simulink model "Example_7"  (R2020b)
settings: Solver=VariableStepAuto  StartTime=0.0  StopTime=0.1  RelTol=1e-3
libraries: fl_lib x10, nesl_utility x4, dspsigops x3, ee_lib x3
settings Model: Creator=zaliyazici  LastModifiedBy=zaliyazici

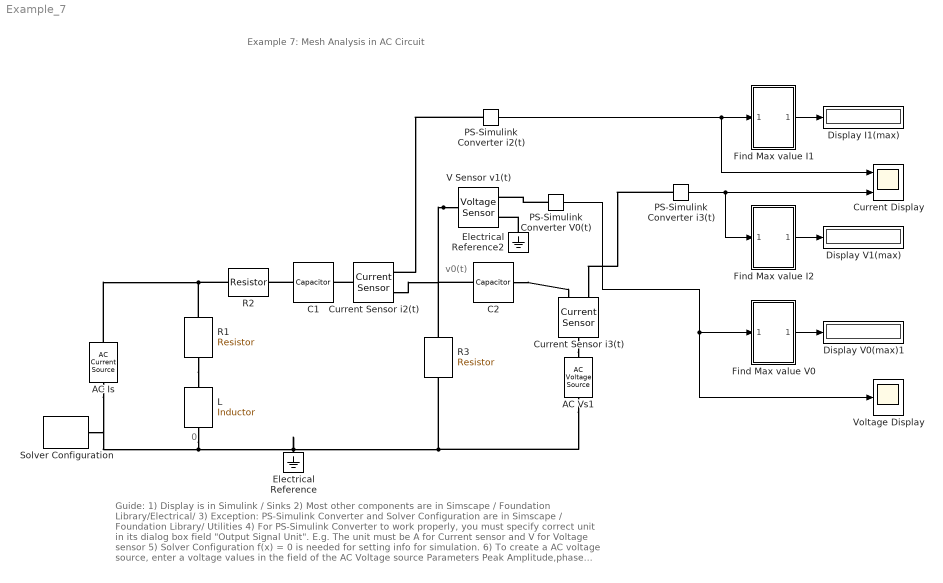
== system Example_7 ==
  note: Guide:
      | 1) Display is in Simulink / Sinks
      | 2) Most other components are in Simscape / Foundation Library/Electrical/
      | 3) Exception: PS-Simulink Converter and Solver Configuration are in Simscape / Foundation Library/ Utilities
      | 4) For PS-Simulink Converter to work properly, you must specify correct unit in its dialog box field "Output Signal Unit".
      | E.g. The unit must be A for Current sensor and V for Voltage sensor
      | 5) Solver Configuration f(x) = 0 is needed for setting info for simulation.
      | 6) To create a AC voltage source, enter a voltage values in the field of the AC Voltage source Parameters Peak Amplitude,phase shift and Frequency. Use 90 degree in phase o conver cosine signal.
      | 7) To create "Annotation", double-click a location on project page and select "Create annotation" from the prompt. Then, type any text you want to clarify your circuit. E.g. "Display for Current".
      | 8) To understand how to use a component, right-click on the component and select "Help".
      | Measurement: Current $i_2(t), i_3(t)$ , and voltage $v_0(t)$
  note: Example 7: Mesh Analysis in AC Circuit
  note: 0
  note: v0(t)
  AC Is : fl_lib/Electrical/Electrical Sources/AC Current Source  amp=200 mA  shift=90 deg  frequency=60 Hz  omega=0 rad/s
      settings: SourceProductBaseCode=SS  InternalSimscapePortConfiguration="{\"Bottom\":[],\"Left\":[{\"id\":\"p\",\"label\":\"\",\"type\":\"foundation.electrical.electrical\"}],\"Right\":[{\"id\":\"n\",\"label\":\"\",\"type\":\"foundation.electrical.electrical\"}],\"Top\":[]}"
      settings: AttributesFormatString=|
      | %<amp> %<amp_unit>
      | %<frequency> %<frequency_unit>
      | %<shift> %<shift_unit>
  AC Vs1 : fl_lib/Electrical/Electrical Sources/AC Voltage Source  amp=36 V  shift=90-45 deg  frequency=60 Hz  omega=0 rad/s
      settings: AttributesFormatString=|
      | %<amp> %<amp_unit>
      | %<frequency> %<frequency_unit>
      | %<shift> %<shift_unit>
  C1 : fl_lib/Electrical/Electrical Elements/Capacitor  c=100 uF  r=1e-6 Ohm  g=0 1/Ohm  i_specify=off  i_priority=None  i=0 A  i_nominal_specify=off  i_nominal_unit=A  i_nominal_value=1  v_specify=off  v_priority=None  v=0 V  v_nominal_specify=off  v_nominal_unit=V  v_nominal_value=1  vc_specify=on  vc_priority=High  vc=0 V  vc_nominal_specify=off  vc_nominal_unit=V  vc_nominal_value=1
      settings: AttributesFormatString=%<c> %<c_unit>
  C2 : fl_lib/Electrical/Electrical Elements/Capacitor  c=200 uF  r=1e-6 Ohm  g=0 1/Ohm  i_specify=off  i_priority=None  i=0 A  i_nominal_specify=off  i_nominal_unit=A  i_nominal_value=1  v_specify=off  v_priority=None  v=0 V  v_nominal_specify=off  v_nominal_unit=V  v_nominal_value=1  vc_specify=on  vc_priority=High  vc=0 V  vc_nominal_specify=off  vc_nominal_unit=V  vc_nominal_value=1
      settings: AttributesFormatString=%<c> %<c_unit>
  Current Display : Scope  NumInputPorts=2
  Current Sensor i2(t) : fl_lib/Electrical/Electrical Sensors/Current Sensor
  Current Sensor i3(t) : fl_lib/Electrical/Electrical Sensors/Current Sensor
  Display I1(max) : Display
  Display V0(max)1 : Display
  Display V1(max) : Display
  Electrical Reference : fl_lib/Electrical/Electrical Elements/Electrical Reference
  Electrical Reference2 : fl_lib/Electrical/Electrical Elements/Electrical Reference
  Find Max value I1 : Subsystem
  Find Max value I2 : Subsystem
  Find Max value V0 : Subsystem
  L : fl_lib/Electrical/Electrical Elements/Inductor  l=100 mH  r=0 Ohm  g=1e-9 1/Ohm  i_specify=off  i_priority=None  i=0 A  i_nominal_specify=off  i_nominal_unit=A  i_nominal_value=1  v_specify=off  v_priority=None  v=0 V  v_nominal_specify=off  v_nominal_unit=V  v_nominal_value=1  i_L_specify=on  i_L_priority=High  i_L=0 mA  i_L_nominal_specify=off  i_L_nominal_unit=A  i_L_nominal_value=1
      settings: AttributesFormatString=%<l> %<l_unit>
  PS-Simulink Converter V0(t) : nesl_utility/PS-Simulink Converter  PhysicalDomain=network_engine_domain  SubClassName=ps_output  LeftPortType=input  RightPortType=output  PseudoPeriodic=off  Frequencies=[]  Unit=V  AffineConversion=off
  PS-Simulink Converter i2(t) : nesl_utility/PS-Simulink Converter  PhysicalDomain=network_engine_domain  SubClassName=ps_output  LeftPortType=input  RightPortType=output  PseudoPeriodic=off  Frequencies=[]  Unit=A  AffineConversion=off
  PS-Simulink Converter i3(t) : nesl_utility/PS-Simulink Converter  PhysicalDomain=network_engine_domain  SubClassName=ps_output  LeftPortType=input  RightPortType=output  PseudoPeriodic=off  Frequencies=[]  Unit=A  AffineConversion=off
  R1 : ee_lib/Passive/Resistor  R=80 Ohm  R_tol=5  enable_R_tol=0  tol_distribution=1  nSigma=4  enable_operating_limits=0  operating_limit_action=2  max_working_voltage=100 V  power_rating=1 W  enable_faults=0  fault_action=1  R_faulted=inf Ohm  enable_temporal_fault=0  t_fault=1 s  enable_behavioral_fault=0  max_permissible_current=1 A  t_fail_on_current=1 s  noise_mode=0  sample_time=1e-3 s  repeatability=1  auto_seed=430448238  user_seed=0  Tdevice=25 degC  alpha=3.93e-3 1/K  Tmeas=25 degC  thermal_mass=100 J/K  power_derating_T1=70 degC  power_derating_T2=155 degC  operating_temperature_range_vec=[-50, 150] degC  temperature_specify=off  temperature_priority=High  temperature=298.15 K  temperature_nominal_specify=off  temperature_nominal_unit=K  temperature_nominal_value=1
      settings: AttributesFormatString=%<R> %<R_unit>
  R2 : ee_lib/Passive/Resistor  R=100 Ohm  R_tol=5  enable_R_tol=0  tol_distribution=1  nSigma=4  enable_operating_limits=0  operating_limit_action=2  max_working_voltage=100 V  power_rating=1 W  enable_faults=0  fault_action=1  R_faulted=inf Ohm  enable_temporal_fault=0  t_fault=1 s  enable_behavioral_fault=0  max_permissible_current=1 A  t_fail_on_current=1 s  noise_mode=0  sample_time=1e-3 s  repeatability=1  auto_seed=57050912  user_seed=0  Tdevice=25 degC  alpha=3.93e-3 1/K  Tmeas=25 degC  thermal_mass=100 J/K  power_derating_T1=70 degC  power_derating_T2=155 degC  operating_temperature_range_vec=[-50, 150] degC  temperature_specify=off  temperature_priority=High  temperature=298.15 K  temperature_nominal_specify=off  temperature_nominal_unit=K  temperature_nominal_value=1
      settings: AttributesFormatString=%<R> %<R_unit>
  R3 : ee_lib/Passive/Resistor  R=200 Ohm  R_tol=5  enable_R_tol=0  tol_distribution=1  nSigma=4  enable_operating_limits=0  operating_limit_action=2  max_working_voltage=100 V  power_rating=1 W  enable_faults=0  fault_action=1  R_faulted=inf Ohm  enable_temporal_fault=0  t_fault=1 s  enable_behavioral_fault=0  max_permissible_current=1 A  t_fail_on_current=1 s  noise_mode=0  sample_time=1e-3 s  repeatability=1  auto_seed=1294739146  user_seed=0  Tdevice=25 degC  alpha=3.93e-3 1/K  Tmeas=25 degC  thermal_mass=100 J/K  power_derating_T1=70 degC  power_derating_T2=155 degC  operating_temperature_range_vec=[-50, 150] degC  temperature_specify=off  temperature_priority=High  temperature=298.15 K  temperature_nominal_specify=off  temperature_nominal_unit=K  temperature_nominal_value=1
      settings: AttributesFormatString=%<R> %<R_unit>
  Solver Configuration : nesl_utility/Solver Configuration  PhysicalDomain=network_engine_domain  SubClassName=solver  LeftPortType=input  RightPortType=generic  Tones=[]  Harmonics=[]  SimulateNoise=off  Profile=off  UseLocalSampling=off  EnableSwitchedLinearOptims=on  FrequencyDomain=off  UseCCode=off  RelTol=0.001  AbsTol=1e-06  MinStep=1e-09  ToWorkspace=off  RevertToSquareIcSolve=off  NumHomotopyIterations=100  PhasorMode=off  PhasorModeNumHarmonics=1  DoDC=off  ResidualTolerance=1e-09  UseLocalSolver=off  LocalSolverChoice=NE_BACKWARD_EULER_ADVANCER  LocalSolverSampleTime=0.001  DoFixedCost=off  MaxNonlinIter=3  MaxModeIter=2  ComputeImpulses=off  ImpulseIterations=2  LinearAlgebra=auto  EquationFormulation=NE_TIME_EF  DelaysMemoryBudget=1024  AutomaticFiltering=on  FilteringTimeConstant=0.001  PartitionStorageMethod=AS_NEEDED  PartitionMemoryBudget=1024  PartitionMethod=ROBUST
  V Sensor v1(t) : fl_lib/Electrical/Electrical Sensors/Voltage Sensor
  Voltage Display : Scope
  wires:
  PS-Simulink Converter i3(t)/1 -> Find Max value I2/1(In1), Current Display/2
  PS-Simulink Converter i2(t)/1 -> Current Display/1, Find Max value I1/1(In1)
  Find Max value I2/1(Out2) -> Display V1(max)/1
  Find Max value I1/1(Out2) -> Display I1(max)/1
  Find Max value V0/1(Out2) -> Display V0(max)1/1
  PS-Simulink Converter V0(t)/1 -> Voltage Display/1, Find Max value V0/1(In1)
  connections:
  PS-Simulink Converter i3(t)/LConn1 -- Current Sensor i3(t)/RConn1
  C1/LConn1 -- R2/RConn1
  R2/LConn1 -- AC Is/LConn1 -- R1/LConn1
  V Sensor v1(t)/LConn1 -- C2/RConn1 -- R3/LConn1 -- Current Sensor i2(t)/RConn2
  R1/RConn1 -- L/LConn1
  Electrical Reference2/LConn1 -- V Sensor v1(t)/RConn2
  PS-Simulink Converter V0(t)/LConn1 -- V Sensor v1(t)/RConn1
  Current Sensor i2(t)/LConn1 -- C1/RConn1
  Current Sensor i3(t)/LConn1 -- AC Vs1/LConn1
  C2/LConn1 -- Current Sensor i3(t)/RConn2
  PS-Simulink Converter i2(t)/LConn1 -- Current Sensor i2(t)/RConn1
  AC Is/RConn1 -- Solver Configuration/RConn1 -- L/RConn1 -- R3/RConn1 -- AC Vs1/RConn1 -- Electrical Reference/LConn1

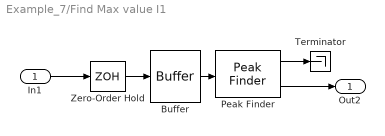
== system Example_7/Find Max value I1 ==
  In1 : Inport
  Buffer : Buffer  N=256  OutputFrames=off
  Peak Finder : dspsigops/Peak Finder  polarity=Maxima  outputIdx=off  outputVal=on  maxPeaks=1  NoiseDistinguish=off  thresh=0  roundingMode=Floor  overflowMode=off
      settings: SourceProductBaseCode=DS  allowOverrides=off
  Terminator : Terminator
  Zero-Order Hold : ZeroOrderHold  SampleTime=1e-4
  Out2 : Outport
  wires:
  Buffer/1 -> Peak Finder/1
  Zero-Order Hold/1 -> Buffer/1
  Peak Finder/2 -> Out2/1
  Peak Finder/1 -> Terminator/1
  In1/1 -> Zero-Order Hold/1

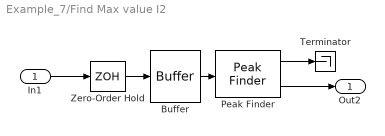
== system Example_7/Find Max value I2 ==
  In1 : Inport
  Buffer : Buffer  N=256  OutputFrames=off
  Peak Finder : dspsigops/Peak Finder  polarity=Maxima  outputIdx=off  outputVal=on  maxPeaks=1  NoiseDistinguish=off  thresh=0  roundingMode=Floor  overflowMode=off
      settings: SourceProductBaseCode=DS  allowOverrides=off
  Terminator : Terminator
  Zero-Order Hold : ZeroOrderHold  SampleTime=1e-4
  Out2 : Outport
  wires:
  Buffer/1 -> Peak Finder/1
  Zero-Order Hold/1 -> Buffer/1
  Peak Finder/2 -> Out2/1
  Peak Finder/1 -> Terminator/1
  In1/1 -> Zero-Order Hold/1

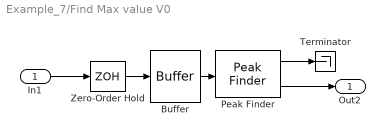
== system Example_7/Find Max value V0 ==
  In1 : Inport
  Buffer : Buffer  N=256  OutputFrames=off
  Peak Finder : dspsigops/Peak Finder  polarity=Maxima  outputIdx=off  outputVal=on  maxPeaks=1  NoiseDistinguish=off  thresh=0  roundingMode=Floor  overflowMode=off
      settings: SourceProductBaseCode=DS  allowOverrides=off
  Terminator : Terminator
  Zero-Order Hold : ZeroOrderHold  SampleTime=1e-4
  Out2 : Outport
  wires:
  Buffer/1 -> Peak Finder/1
  Zero-Order Hold/1 -> Buffer/1
  Peak Finder/2 -> Out2/1
  Peak Finder/1 -> Terminator/1
  In1/1 -> Zero-Order Hold/1
